simulink model "chap14_2"  (Simulink 7.5)
settings: Solver=FixedStepDiscrete  StartTime=0.0  StopTime=0.0  RelTol=1e-3
undefined symbols (not defined in the file): gray
libraries: vipsnks x3, vipsrcs x2, vipanalysis x1
settings Model: Creator=Administrator  LastModifiedBy=Administrator

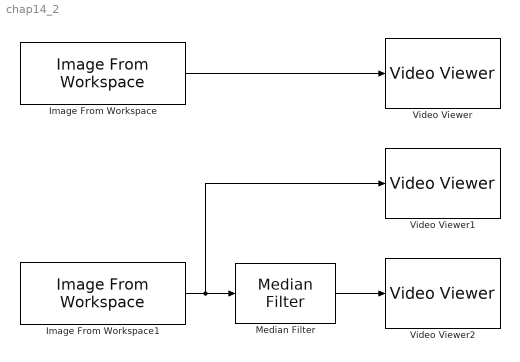
== system chap14_2 ==
  Image From Workspace : vipsrcs/Image From Workspace  Tag=vipblks_nd  SystemSampleTime=-1  ImageValue=A  Ts=inf  imagePorts=One multidimensional signal  ImageDataType=Inherit from 'Value'  Signed=on  WordLength=16  sdImageDataType=sfix(16)  FractionLengthMode=User-defined  FractionLength=15  OutPortLabels=R|G|B
  Image From Workspace1 : vipsrcs/Image From Workspace  Tag=vipblks_nd  SystemSampleTime=-1  ImageValue=B  Ts=inf  imagePorts=One multidimensional signal  ImageDataType=Inherit from 'Value'  Signed=on  WordLength=16  sdImageDataType=sfix(16)  FractionLengthMode=User-defined  FractionLength=15  OutPortLabels=R|G|B
  Median Filter : vipanalysis/Median Filter  DialogController=vipDDGCreate  DialogControllerArgs=DataTag0  nghbood=[3 3]  outSize=Same as input port I  padType=Constant  padSrc=Specify via dialog  padVal=0  roundingMode=Floor  overflowMode=off
  Video Viewer : vipsnks/Video Viewer  DialogControllerArgs=DataTag2  inputType=Obsolete7b  imagePorts=One multidimensional signal  useColorMap=off  colormapValue=gray(256)  specRange=off  minInputVal=0  maxInputVal=255  FigPos=[152 486 410 300]  AxisZoom=on  trueSizedOnce=off  OpenAtMdlStart=on
  Video Viewer1 : vipsnks/Video Viewer  DialogControllerArgs=DataTag4  inputType=Obsolete7b  imagePorts=One multidimensional signal  useColorMap=off  colormapValue=gray(256)  specRange=off  minInputVal=0  maxInputVal=255  FigPos=[755 573 410 300]  AxisZoom=on  trueSizedOnce=off  OpenAtMdlStart=on
  Video Viewer2 : vipsnks/Video Viewer  DialogControllerArgs=DataTag6  inputType=Obsolete7b  imagePorts=One multidimensional signal  useColorMap=off  colormapValue=gray(256)  specRange=off  minInputVal=0  maxInputVal=255  FigPos=[14 857 410 300]  AxisZoom=on  trueSizedOnce=off  OpenAtMdlStart=on
  wires:
  Image From Workspace/1 -> Video Viewer/1
  Image From Workspace1/1 -> Median Filter/1, Video Viewer1/1
  Median Filter/1 -> Video Viewer2/1
